simulink model "host_cam_robot_demo"  (Simulink 7.3)
settings: Solver=ode45  StartTime=0.0  StopTime=inf  RelTol=1e-3
undefined symbols (not defined in the file): gray
libraries: vipsnks x2, waijung_socket_lib x2, simulink x2, waijung_image_sensor_lib x1
settings Model: Creator=Krisada  LastModifiedBy=Krisada

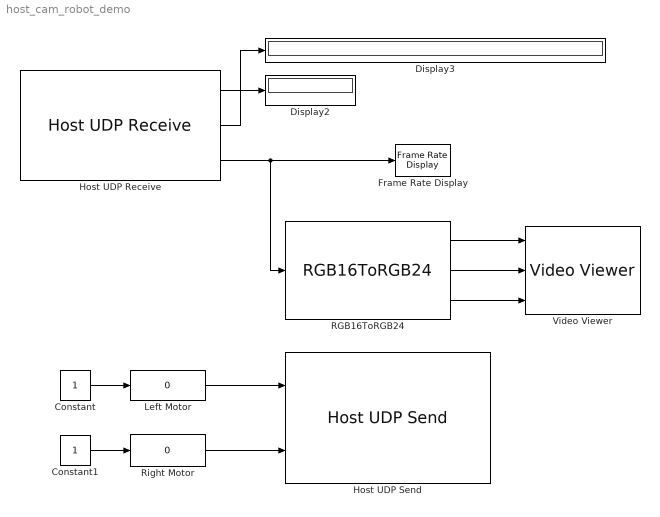
== system host_cam_robot_demo ==
  Constant : Constant  OutDataType=fixdt(1, 16)  OutScaling=2^0
  Constant1 : Constant  OutDataType=fixdt(1, 16)  OutScaling=2^0
  Display2 : Display
  Display3 : Display
  Frame Rate Display : vipsnks/Frame Rate Display  DialogController=vipDDGCreate  DialogControllerArgs=DataTag0  UpdateRate=10
  Host UDP Receive : waijung_socket_lib/Host UDP Receive  conf=HostReceive  protocol=UDP  port=7  address=192.168.1.21  echo=off  transfer=Blocking  timeout=5  datasource=BufferStream  datatype=uint16  datacount=120*160  porttype_double=0  porttype_single=0  porttype_int8=0  porttype_uint8=0  porttype_int16=0  porttype_uint16=0  porttype_int32=0  porttype_uint32=1  portpinstr=0  sampletime=0.01  blockid=HostUDPReceive  inputporttype=[]  inputportwidth=[]  inputportlabel={}  outputporttype=[5,3,5]  outputportwidth=[1,4,19200]  outputportlabel={'Remote Port','Remote IP(1:4)','Data(1:19200)'}  compat=0  optionstring=[]  options=[7,2,1,5000,1]
  Host UDP Send : waijung_socket_lib/Host UDP Send  conf=HostSend  protocol=UDP  variableipport=off  port=7  address=192.168.1.31  echo=off  transfer=Blocking  timeout=5  datasource=Ports  datatype=uint8  datacount=2  porttype_double=2  porttype_single=0  porttype_int8=0  porttype_uint8=0  porttype_int16=0  porttype_uint16=0  porttype_int32=0  porttype_uint32=0  portpinstr=0  sampletime=0.1  blockid=HostUDPSend  inputporttype=[0,0]  inputportwidth=[1]  inputportlabel={'D0 double','D1 double'}  outputporttype=[]  outputportwidth=[]  outputportlabel={}  compat=0  optionstring=[]  options=[7,2,0,5000,0]
  Left Motor : simulink/Math Operations/Slider Gain  SystemSampleTime=-1  low=-100  gain=0  high=100
  RGB16ToRGB24 : waijung_image_sensor_lib/RGB16ToRGB24  conf=RGB16ToRGB24  column=120  row=160  inputalignment=RGB  outputalignment=BGR  colorseparate=on  simparams=[0 160 0 1]  portpinstr=0  sampletime=-1  blockid=RGB16ToRGB24  inputporttype=[5]  inputportwidth=[19200]  inputportlabel={'Input'}  outputporttype="[3  3 3]"  outputportwidth=[120 120 120]  outputportlabel={'B','G','R'}  compat=0  optionstring=[]
  Right Motor : simulink/Math Operations/Slider Gain  SystemSampleTime=-1  low=-100  gain=0  high=100
  Video Viewer : vipsnks/Video Viewer  DialogControllerArgs=DataTag2  inputType=Obsolete7b  imagePorts=Separate color signals  useColorMap=off  colormapValue=gray(256)  specRange=off  minInputVal=0  maxInputVal=255  FigPos=[194 953 480 382]  AxisZoom=on  trueSizedOnce=off  OpenAtMdlStart=on
  wires:
  Host UDP Receive/3 -> RGB16ToRGB24/1, Frame Rate Display/1
  Host UDP Receive/1 -> Display2/1
  Host UDP Receive/2 -> Display3/1
  RGB16ToRGB24/2 -> Video Viewer/2
  RGB16ToRGB24/3 -> Video Viewer/3
  RGB16ToRGB24/1 -> Video Viewer/1
  Constant/1 -> Left Motor/1
  Constant1/1 -> Right Motor/1
  Left Motor/1 -> Host UDP Send/1
  Right Motor/1 -> Host UDP Send/2
